simulink model "BWS_discrete_PIDF"  (R2023b)
settings: Solver=VariableStepAuto  StartTime=0.0  StopTime=40.0  RelTol=1e-3
values from neighbouring files (symbols this model uses):
  A = [0,-r/(2*J),0;k*r/2,0,-k/2;0,1/(2*m),0]    [discrete_pidf_bws.m]
  B = [1/J,0;0,0;0,1/m]    [discrete_pidf_bws.m]
  BTI = .005    (= 0.005)    [discrete_pidf_bws.m]
  C2 = [1,0,0;0,1,0;0,0,1]    [discrete_pidf_bws.m]
  D2 = [0,0;0,0;0,0]    [discrete_pidf_bws.m]
  g = 9.81    [discrete_pidf_bws.m]
  ka = .41    (= 0.41)    [discrete_pidf_bws.m]
  km = .0507    (= 0.0507)    [discrete_pidf_bws.m]
  m = 1    [discrete_pidf_bws.m]
  N = 5.9    [discrete_pidf_bws.m]
  x0 = [0, 0, 0]    [discrete_pidf_bws.m]
libraries: slpidlib x1
settings Model: Creator=evere  LastModifiedBy=evere

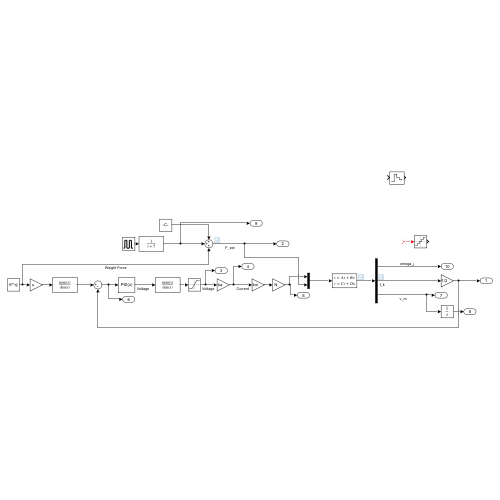
[thumbnail: Simulink's stored preview of the top-level diagram]
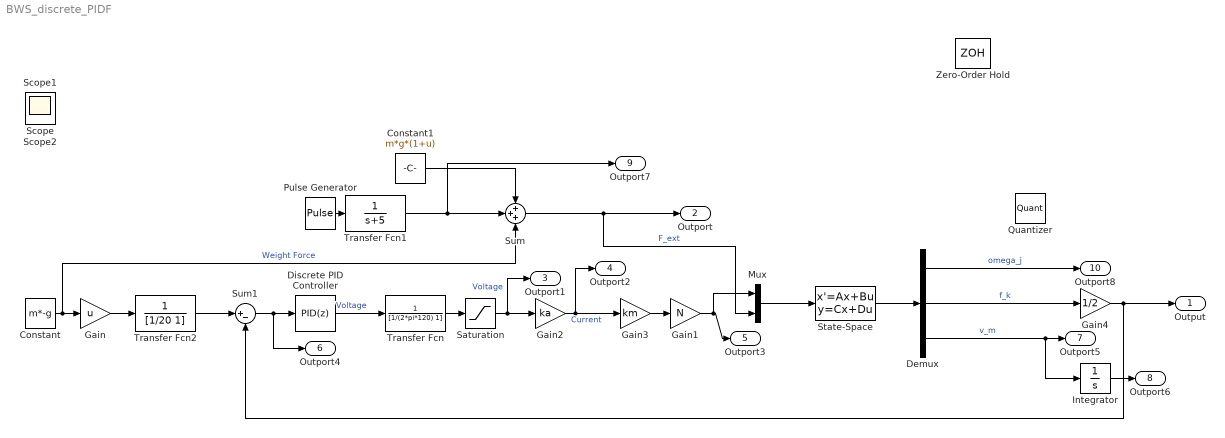
== system BWS_discrete_PIDF ==
  Constant : Constant  Value=m*-g
  Constant1 : Constant  Value=m*g*(1+u)
  Demux : Demux  Outputs=3
  Discrete PID Controller : slpidlib/PID Controller  Controller=PID  Form=Parallel  TimeDomain=Discrete-time  UseExternalTs=off  SampleTime=.0001  IntegratorMethod=Forward Euler  FilterMethod=Forward Euler  ControllerParametersSource=internal  P=0.949201655564499  I=11.0489075266223  UseKiTs=off  D=0.0198521148315682  N=7725.96987053356  UseFilter=on  TunerSelectOption=Transfer Function Based (PID Tuner App)  InitialConditionSource=internal  InitialConditionForIntegrator=0  InitialConditionForFilter=0  DifferentiatorICPrevScaledInput=0  ExternalReset=none  TrackingMode=off  Kt=1  LimitOutput=off  SatLimitsSource=internal  UpperSaturationLimit=inf  LowerSaturationLimit=-inf  LinearizeAsGain=off  AntiWindupMode=none  Kb=1  LimitIntegrator=off  UpperIntegratorSaturationLimit=inf  LowerIntegratorSaturationLimit=-inf  POutMin=[]  POutMax=[]  IOutMin=[]  IOutMax=[]  DOutMin=[]  DOutMax=[]  NOutMin=[]  NOutMax=[]  SumOutMin=[]  SumOutMax=[]  SaturationOutMin=[]  SaturationOutMax=[]  PParamMin=[]  PParamMax=[]  IParamMin=[]  IParamMax=[]  DParamMin=[]  DParamMax=[]  NParamMin=[]  NParamMax=[]  KbParamMin=[]  KbParamMax=[]  KtParamMin=[]  KtParamMax=[]  KbOutMin=[]  KbOutMax=[]  KtOutMin=[]  KtOutMax=[]  IntegratorOutMin=[]  IntegratorOutMax=[]  FilterOutMin=[]  FilterOutMax=[]  SumI1OutMin=[]  SumI1OutMax=[]  SumI2OutMin=[]  SumI2OutMax=[]  SumI3OutMin=[]  SumI3OutMax=[]  SumI4OutMin=[]  SumI4OutMax=[]  SumDOutMin=[]  SumDOutMax=[]  DifferentiatorOutMin=[]  DifferentiatorOutMax=[]  FilterDiffOutCoefMin=[]  FilterDiffOutCoefMax=[]  ReciprocalOutMin=[]  ReciprocalOutMax=[]  SumDenOutMin=[]  SumDenOutMax=[]  SumNumOutMin=[]  SumNumOutMax=[]  DivideOutMin=[]  DivideOutMax=[]  UdiffTsProdOutMin=[]  UdiffTsProdOutMax=[]  NTsProdOutMin=[]  NTsProdOutMax=[]  UintegralTsProdOutMin=[]  UintegralTsProdOutMax=[]  UngainTsProdOutMin=[]  UngainTsProdOutMax=[]  ClampingZeroOutDataTypeStr=Inherit: Inherit via back propagation  ClampingZeroOutMin=[]  ClampingZeroOutMax=[]  FilterDenConstantOutDataTypeStr=Inherit: Inherit via back propagation  FilterDenConstantOutMin=[]  FilterDenConstantOutMax=[]  PCopyOutDataTypeStr=Inherit: Inherit via back propagation  PCopyOutMin=[]  PCopyOutMax=[]  NCopyOutDataTypeStr=Inherit: Inherit via back propagation  NCopyOutMin=[]  NCopyOutMax=[]  IntegratorContinuousStateAttributes=''  IntegratorStateMustResolveToSignalObject=off  IntegratorRTWStateStorageClass=Auto  FilterContinuousStateAttributes=''  FilterStateMustResolveToSignalObject=off  FilterRTWStateStorageClass=Auto  ParallelPVariant=InternalParameters  IdealPVariant=Disabled  IVariant=InternalParameters  DVariant=InternalParameters  IntegratorVariant=Discrete  SatVariant=Disabled  AWVariant=Passthrough  PCopyVariant=Disabled  TRVariant=Disabled  FdbkBlocksVariant=Forward  IdealPFdbkVariant=Disabled  SatFdbkVariant=Disabled  DerivativeFilterVariant=ForwardEulerFilter  NVariant=InternalParameters  NCopyVariant=Disabled  FilterICVariant=InternalICsFilter  IntegratorICVariant=InternalICs  ExternalResetVariant=Disabled  TRSumVariant=Passthrough  SumFdbkVariant=Disabled  SumVariant=Sum_PID  TsampFilterVariant=InternalTs  TsampNgainVariant=Passthrough  TsampIntegralVariant=Disabled_SignalSpec  ExternalSaturationOutDataTypeStr=Inherit: Same as second input
      settings: LibrarySourceBlock=simulink/Discrete/Discrete PID Controller
  Gain : Gain  Gain=u
  Gain1 : Gain  Gain=N
  Gain2 : Gain  Gain=ka
  Gain3 : Gain  Gain=km
  Gain4 : Gain  Gain=1/2
  Integrator : Integrator
  Mux : Mux  Inputs=2
  Pulse Generator : DiscretePulseGenerator  PulseType=Time based  Amplitude=5  Period=10  PulseWidth=30
  Quantizer : Quantizer  QuantizationInterval=.0126
  Saturation : Saturate  UpperLimit=7.5  LowerLimit=-7.5
  State-Space : StateSpace  A=A  B=B  C=C2  D=D2  InitialCondition=x0
  Sum : Sum  Inputs=+++
  Sum1 : Sum  Inputs=|+-
  Transfer Fcn : TransferFcn  Denominator=[1/(2*pi*120) 1]
  Transfer Fcn1 : TransferFcn  Denominator=[1 5]
  Transfer Fcn2 : TransferFcn  Denominator=[1/20 1]
  Zero-Order Hold : ZeroOrderHold  SampleTime=BTI
  Output : Outport
  Outport : Outport  Port=2
  Outport1 : Outport  Port=3
  Outport2 : Outport  Port=4
  Outport3 : Outport  Port=5
  Outport4 : Outport  Port=6
  Outport5 : Outport  Port=7
  Outport6 : Outport  Port=8
  Outport7 : Outport  Port=9
  Outport8 : Outport  Port=10
  Scope : Scope
  Scope1 : Scope
  Scope2 : Scope
  wires:
  Constant/1 -> Gain/1, Sum/3  "Weight Force"
  Sum/1 -> Mux/2, Outport/1  "F_ext"
  Discrete PID Controller/1 -> Transfer Fcn/1  "Voltage"
  Gain3/1 -> Gain1/1
  Gain2/1 -> Outport2/1, Gain3/1  "Current"
  Gain1/1 -> Mux/1, Outport3/1
  Mux/1 -> State-Space/1
  State-Space/1 -> Demux/1
  Demux/1 -> Outport8/1  "omega_j"
  Demux/3 -> Integrator/1, Outport5/1  "v_m"
  Gain/1 -> Transfer Fcn2/1
  Sum1/1 -> Discrete PID Controller/1, Outport4/1
  Integrator/1 -> Outport6/1
  ? -> Quantizer/1
  Demux/2 -> Gain4/1  "f_k"
  Pulse Generator/1 -> Transfer Fcn1/1
  Transfer Fcn1/1 -> Outport7/1, Sum/2
  Gain4/1 -> Sum1/2, Output/1
  Constant1/1 -> Sum/1
  Transfer Fcn/1 -> Saturation/1
  Saturation/1 -> Outport1/1, Gain2/1  "Voltage"
  Transfer Fcn2/1 -> Sum1/1
